simulink model "NPNV_CSAD_model"  (R2017a)
settings: Solver=ode4  StartTime=0.0  StopTime=t_sim  FixedStep=0.01  RelTol=1e-3
values from neighbouring files (symbols this model uses):
  eta_initial = [5; -1; 0]    [Run4corner.m]    (also in Simulation_plot.m = [-4; -2; 0.6*pi])
  gamma = 1.5    [Run4corner.m]
  nu_initial = [0; 0; 0]    [Run4corner.m]    (also in Simulation_plot.m)
  sigma = 2    [Run4corner.m]
undefined symbols (not defined in the file or in its folder): fdesignblkfcn, gcbh
libraries: simulink x4, dsparch4 x1
settings Model: Creator=torees  LastModifiedBy=torees

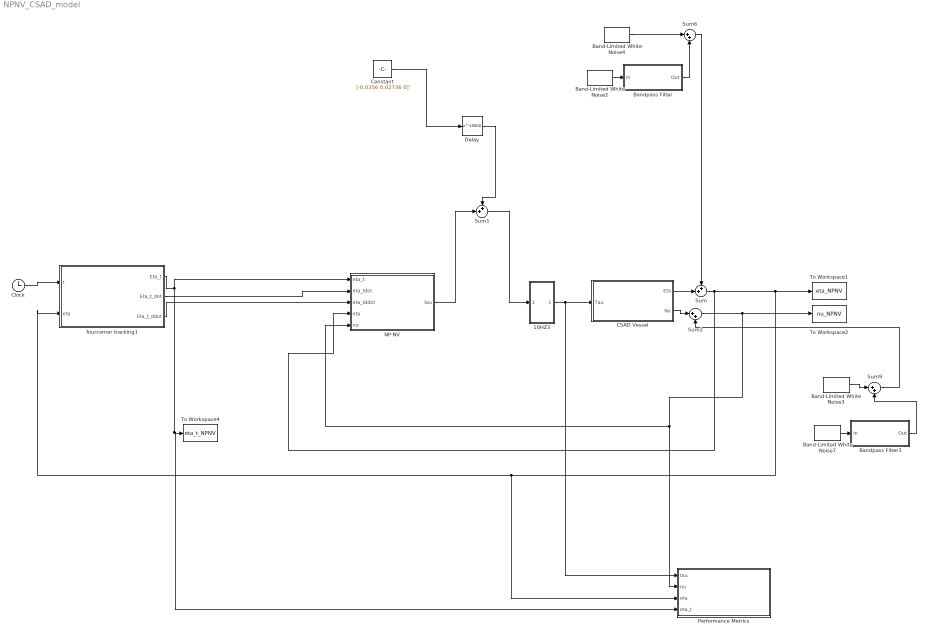
== system NPNV_CSAD_model ==
  10HZ3 : Subsystem
  Band-Limited White Noise2 : simulink/Sources/Band-Limited White Noise  Cov=posnoise  Ts=0.01  seed=[233451]
  Band-Limited White Noise3 : simulink/Sources/Band-Limited White Noise  Cov=velnoise2  Ts=0.01  seed=[233451]
  Band-Limited White Noise4 : simulink/Sources/Band-Limited White Noise  Cov=posnoise2  Ts=0.01  seed=[233451]
  Band-Limited White Noise7 : simulink/Sources/Band-Limited White Noise  Cov=velnoise  Ts=0.01  seed=[23345]
  Bandpass Filter : Subsystem  DialogController=fdesignblkfcn  InitFcn=fdesignblkfcn(gcbh, {'InitFcn'});  mask(Bandpass Filter){}
      mask help: Design a bandpass filter
      settings: CopyFcn=fdesignblkfcn(gcbh, {'CopyFcn'});
      mask Help: helpview(mapfilelocation('dsp'), 'dspbandpassfilter');
      mask Display: disp('Bandpass');
  Bandpass Filter3 : Subsystem  DialogController=fdesignblkfcn  InitFcn=fdesignblkfcn(gcbh, {'InitFcn'});  mask(Bandpass Filter){}
      mask help: Design a bandpass filter
      settings: CopyFcn=fdesignblkfcn(gcbh, {'CopyFcn'});
      mask Help: helpview(mapfilelocation('dsp'), 'dspbandpassfilter');
      mask Display: disp('Bandpass');
  CSAD Vessel : Subsystem
  Clock : Clock
  Constant : Constant  Value=[-0.0356 0.02736 0]'
  Delay : Delay  DelayLength=15000  InitialCondition=0
  NP-NV : Subsystem
  "Performance Metrics " : Subsystem
  Sum : Sum  Inputs=++|
  Sum1 : Sum  Inputs=++|
  Sum2 : Sum  Inputs=|++
  Sum6 : Sum  Inputs=|++
  Sum9 : Sum  Inputs=|++
  To Workspace1 : ToWorkspace  VariableName=eta_NPNV  SampleTime=-1
  To Workspace2 : ToWorkspace  VariableName=nu_NPNV  SampleTime=-1
  To Workspace4 : ToWorkspace  VariableName=eta_t_NPNV  SampleTime=-1
  fourcorner tracking1 : MATLAB Function  TreatAsAtomicUnit=on
  wires:
  Clock/1 -> fourcorner tracking1/1(t)
  Sum1/1 -> 10HZ3/1(In1)
  10HZ3/1(Out1) -> "Performance Metrics "/1(tau), CSAD Vessel/1(Tau)
  fourcorner tracking1/1(Eta_t) -> "Performance Metrics "/4(eta_t), To Workspace4/1, NP-NV/1(eta_t)
  fourcorner tracking1/2(Eta_t_dot) -> NP-NV/2(eta_tdot)
  fourcorner tracking1/3(Eta_t_ddot) -> NP-NV/3(eta_tddot)
  Sum6/1 -> Sum/1
  CSAD Vessel/1(Eta) -> Sum/2
  Sum/1 -> "Performance Metrics "/3(eta), fourcorner tracking1/2(eta), To Workspace1/1, NP-NV/4(eta)
  Delay/1 -> Sum1/1
  NP-NV/1(tau) -> Sum1/2
  CSAD Vessel/2(Nu) -> Sum2/1
  Sum9/1 -> Sum2/2
  Sum2/1 -> NP-NV/5(nu), "Performance Metrics "/2(nu), To Workspace2/1
  Constant/1 -> Delay/1
  Band-Limited White Noise2/1 -> Bandpass Filter/1(In)
  Band-Limited White Noise4/1 -> Sum6/1
  Bandpass Filter/1(Out) -> Sum6/2
  Bandpass Filter3/1(Out) -> Sum9/2
  Band-Limited White Noise3/1 -> Sum9/1
  Band-Limited White Noise7/1 -> Bandpass Filter3/1(In)

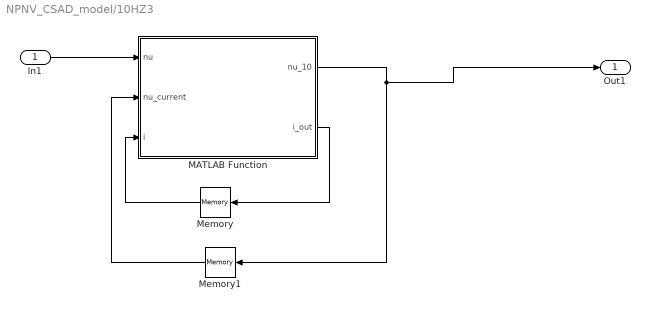
== system NPNV_CSAD_model/10HZ3 ==
  In1 : Inport
  MATLAB Function : MATLAB Function  TreatAsAtomicUnit=on
  Memory : Memory
  Memory1 : Memory
  Out1 : Outport
  wires:
  In1/1 -> MATLAB Function/1(nu)
  MATLAB Function/1(nu_10) -> Memory1/1, Out1/1
  Memory1/1 -> MATLAB Function/2(nu_current)
  MATLAB Function/2(i_out) -> Memory/1
  Memory/1 -> MATLAB Function/3(i)

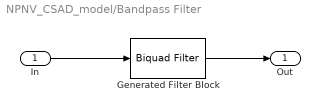
== system NPNV_CSAD_model/Bandpass Filter ==
  In : Inport
  Generated Filter Block : dsparch4/Biquad Filter  Tag=BlockMethodSubSystem  IIRFiltStruct=Direct form II  CoeffSource=Specify via dialog  BiQuadCoeffs=[0.28932621448050977 -0.19800857833013893 0.28932621448050977 1 -0.62679229449728924 0.99326477861490148;2 -1.1003519967587603 2 1 -0.60508947521969358 0.99323977127646146]  a0Flag=Warning  IC=0  ICnum=0  ICden=0  denAccumFracLength=30  denProdOutputFracLength=30  secondMemoryFracLength=15  roundingMode=Floor  overflowMode=off  ScaleValues=[0.0063942944592789474;1;8.4992509081585865]  optimizeScaleValues=off  ScaleValueMode=Specify via input port (g)  scaleValueFracLength=14  FilterSource=Specify via dialog  FilterObject=BQF
      settings: SourceProductName=DSP System Toolbox
  Out : Outport
  wires:
  In/1 -> Generated Filter Block/1
  Generated Filter Block/1 -> Out/1

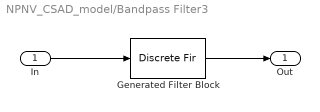
== system NPNV_CSAD_model/Bandpass Filter3 ==
  In : Inport
  Generated Filter Block : DiscreteFir  Tag=BlockMethodSubSystem  Coefficients=[-0.00079916321459414256 0.00032403449583075965 0.0011103641181887203 0.00036251169928540301 -0.0010006208701309827 -0.0010529558624241767 0.00042247970506665205 0.0014337707539335287 0.00046392998912194242 -0.0012699771729577363 -0.0013261148515873755 0.00052825480198556642 0.0017806682220775237 0.00057253310721010274 -0.0015579403216620623 -0.0016176685166059228 0.00064097161479369062 0.0021497454476688454 0.00068789900070729702 -0.0018633612906794794 -0.001926423966618558 0.00076015783376762245 0.0025394203872170606 0.00080952232829501457 -0.0021848742766087973 -0.0022509729150716933 0.00088525944440233741 0.0029478485691564844 0.00093681730481494862 -0.0025209046819104023 -0.0025897001978467645 0.0010156441843386106 0.0033729349354923851 0.0010691215618221929 -0.0028696797458744754 -0.0029407949247964556 0.0011506060003265994 0.003812348898990897 0.0012057009948789105 -0.0032292417393970374 -0.0033022641741789404 0.0012893704679716328 0.0042635424867300802 0.0013457555550174948 -0.0035974636052109902 -0.0036719491047843252 0.0014311011238421125 0.0047237713985051914 0.0014884259288208323 -0.0039720668915110471 -0.0040475433271385287 0.0015749066468750648 0.0051901187680907018 0.0016328010391898516 -0.0043506417948832978 -0.0044266133435287595 0.0017198488140888818 0.0056595213772874303 0.0017779262872743499 -0.0047306690985537492 -0.0048066208371846924 0.0018649511445690331 0.0061287980375845435 0.0019228124454002008 -0.0051095437646606241 -0.0051849465642018798 0.0020092081356957846 0.006594679822660582 0.0020664451012924151 -0.0054845999149232246 -0.0055589155781061344 0.0021515949867898466 0.0070538418073091422 0.00220779454561572 -0.0058531369131032737 -0.0059258234966891535 0.0022910776978809157 0.007502935945119746 0.0023458259879516803 -0.0062124462453399905 -0.0062829635042002249 0.0024266234252861554 0.0079386246987328078 0.0024795099809151538 -0.0065598388810737601 -0.0066276537694263263 0.0025572109712026269 0.0083576150230118152 0.0026078329282708682 -0.0068926727880481882 -0.0069572649518199582 0.002681841281647562 0.0087566922932573402 0.0027298075507009036 -0.007208380269975662 -0.0072692474638047866 0.0027995478258770264 0.0091327537677777949 0.0028444831823420526 -0.0075044947949431794 -0.0075611581577669394 0.0029094067308983286 0.0094828411767955405 0.0029509557723789931 -0.0077786769865693843 -0.0078306861110607664 0.0030105465468665557 0.0098041720378108516 0.0030483774688243128 -0.0080287394582629224 -0.0080756771915687642 0.0031021575230111413 0.010094169311068033 0.0031359656661302583 -0.0082526701835870051 -0.0082941570998561007 0.0031835002792112198 0.010350489027525429 0.0032130114043830301 -0.0084486541125467305 -0.0084843526015811205 0.0032539137653757461 0.010571045545472292 0.0032788870154664479 -0.0086150927643738641 -0.0086447106853366346 0.0033128224092882838 0.010754034120360252 0.0033330529206425396 -0.0087506215518108801 -0.0087739154062236469 0.0033597423634324232 0.010897950505146132 0.0033750634943581687 -0.0088541246196704986 -0.0088709022038571377 0.003394286772396473 0.011001607335037392 0.003404571920619809 -0.0089247470111965682 -0.008934869514801146 0.0034161699946112351 0.011064147090502434 0.0034213339808147739 -0.0089619040090547896 -0.0089652875331887021 0.003425210725237336 0.011085051475196808 0.003425210725237336 -0.0089652875331887021 -0.0089619040090547896 0.0034213339808147739 0.011064147090502434 0.0034161699946112351 -0.008934869514801146 -0.0089247470111965682 0.003404571920619809 0.011001607335037392 0.003394286772396473 -0.0088709022038571377 -0.0088541246196704986 0.0033750634943581687 0.010897950505146132 0.0033597423634324232 -0.0087739154062236469 -0.0087506215518108801 0.0033330529206425396 0.010754034120360252 0.0033128224092882838 -0.0086447106853366346 -0.0086150927643738641 0.0032788870154664479 0.010571045545472292 0.0032539137653757461 -0.0084843526015811205 -0.0084486541125467305 0.0032130114043830301 0.010350489027525429 0.0031835002792112198 ...(+2603 chars)]  InputProcessing=Columns as channels (frame based)
  Out : Outport
  wires:
  In/1 -> Generated Filter Block/1
  Generated Filter Block/1 -> Out/1

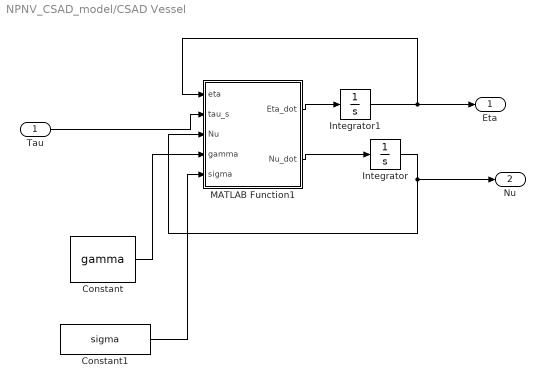
== system NPNV_CSAD_model/CSAD Vessel ==
  Tau : Inport
  Constant : Constant  Value=gamma
  Constant1 : Constant  Value=sigma
  Integrator : Integrator  InitialCondition=nu_initial
  Integrator1 : Integrator  InitialCondition=eta_initial
  MATLAB Function1 : MATLAB Function  TreatAsAtomicUnit=on
  Eta : Outport
  Nu : Outport  Port=2
  wires:
  Integrator/1 -> Nu/1, MATLAB Function1/3(Nu)
  MATLAB Function1/1(Eta_dot) -> Integrator1/1
  Integrator1/1 -> Eta/1, MATLAB Function1/1(eta)
  MATLAB Function1/2(Nu_dot) -> Integrator/1
  Tau/1 -> MATLAB Function1/2(tau_s)
  Constant1/1 -> MATLAB Function1/5(sigma)
  Constant/1 -> MATLAB Function1/4(gamma)

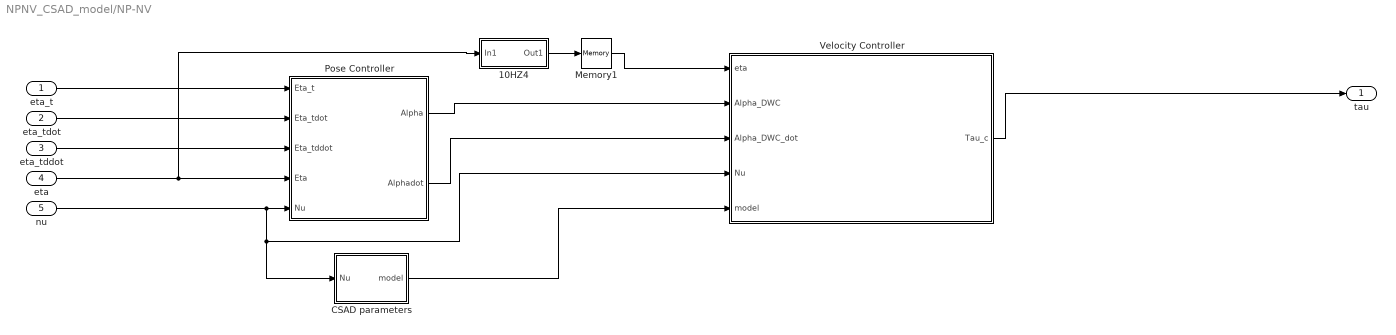
== system NPNV_CSAD_model/NP-NV ==
  eta_t : Inport
  eta_tdot : Inport  Port=2
  eta_tddot : Inport  Port=3
  eta : Inport  Port=4
  nu : Inport  Port=5
  " Pose Controller" : MATLAB Function  TreatAsAtomicUnit=on
  10HZ4 : Subsystem
  CSAD parameters : MATLAB Function  TreatAsAtomicUnit=on
  Memory1 : Memory  X0=[ 0 0 0]'
  Velocity Controller : MATLAB Function  TreatAsAtomicUnit=on
  tau : Outport
  wires:
  eta_t/1 -> " Pose Controller"/1(Eta_t)
  eta_tdot/1 -> " Pose Controller"/2(Eta_tdot)
  eta_tddot/1 -> " Pose Controller"/3(Eta_tddot)
  eta/1 -> 10HZ4/1(In1), " Pose Controller"/4(Eta)
  nu/1 -> Velocity Controller/4(Nu), CSAD parameters/1(Nu), " Pose Controller"/5(Nu)
  CSAD parameters/1(model) -> Velocity Controller/5(model)
  " Pose Controller"/2(Alphadot) -> Velocity Controller/3(Alpha_DWC_dot)
  " Pose Controller"/1(Alpha) -> Velocity Controller/2(Alpha_DWC)
  Velocity Controller/1(Tau_c) -> tau/1
  10HZ4/1(Out1) -> Memory1/1
  Memory1/1 -> Velocity Controller/1(eta)

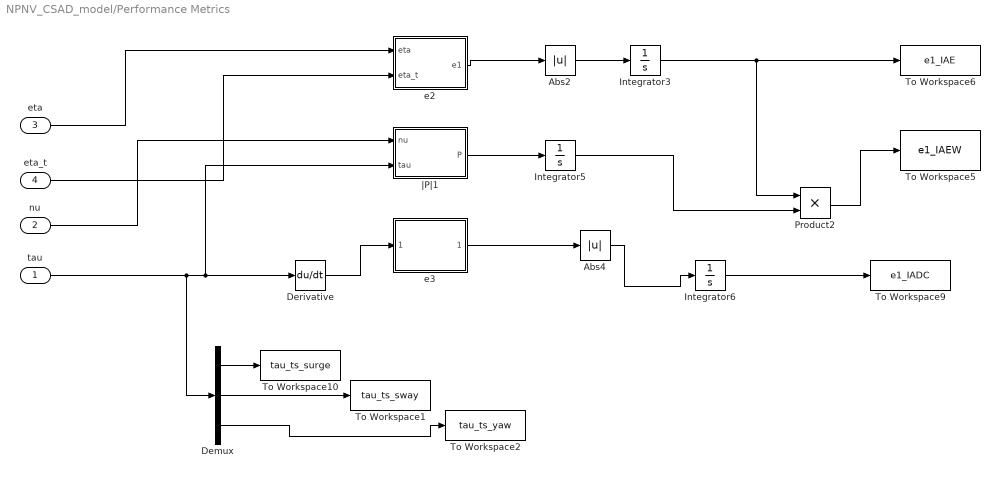
== system NPNV_CSAD_model/Performance Metrics  ==
  tau : Inport
  nu : Inport  Port=2
  eta : Inport  Port=3
  eta_t : Inport  Port=4
  Abs2 : Abs
  Abs4 : Abs
  Demux : Demux  Outputs=3
  Derivative : Derivative
  Integrator3 : Integrator
  Integrator5 : Integrator
  Integrator6 : Integrator
  Product2 : Product
  To Workspace1 : ToWorkspace  VariableName=tau_ts_sway  SaveFormat=Timeseries  SampleTime=-1
  To Workspace10 : ToWorkspace  VariableName=tau_ts_surge  SaveFormat=Timeseries  SampleTime=-1
  To Workspace2 : ToWorkspace  VariableName=tau_ts_yaw  SaveFormat=Timeseries  SampleTime=-1
  To Workspace5 : ToWorkspace  VariableName=e1_IAEW  SaveFormat=Timeseries  SampleTime=-1
  To Workspace6 : ToWorkspace  VariableName=e1_IAE  SaveFormat=Timeseries  SampleTime=-1
  To Workspace9 : ToWorkspace  VariableName=e1_IADC  SaveFormat=Timeseries  SampleTime=-1
  e2 : MATLAB Function  TreatAsAtomicUnit=on
  e3 : MATLAB Function  TreatAsAtomicUnit=on
  |P|1 : MATLAB Function  TreatAsAtomicUnit=on
  wires:
  eta_t/1 -> e2/2(eta_t)
  eta/1 -> e2/1(eta)
  nu/1 -> |P|1/1(nu)
  tau/1 -> Demux/1, |P|1/2(tau), Derivative/1
  Integrator3/1 -> Product2/1, To Workspace6/1
  |P|1/1(P) -> Integrator5/1
  e2/1(e1) -> Abs2/1
  e3/1(tau_dot) -> Abs4/1
  Abs2/1 -> Integrator3/1
  Derivative/1 -> e3/1(tau_dot_in)
  Integrator6/1 -> To Workspace9/1
  Integrator5/1 -> Product2/2
  Product2/1 -> To Workspace5/1
  Abs4/1 -> Integrator6/1
  Demux/1 -> To Workspace10/1
  Demux/2 -> To Workspace1/1
  Demux/3 -> To Workspace2/1

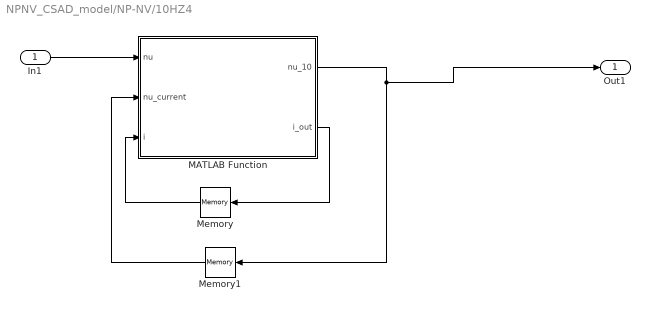
== system NPNV_CSAD_model/NP-NV/10HZ4 ==
  In1 : Inport
  MATLAB Function : MATLAB Function  TreatAsAtomicUnit=on
  Memory : Memory
  Memory1 : Memory
  Out1 : Outport
  wires:
  In1/1 -> MATLAB Function/1(nu)
  MATLAB Function/1(nu_10) -> Memory1/1, Out1/1
  Memory1/1 -> MATLAB Function/2(nu_current)
  MATLAB Function/2(i_out) -> Memory/1
  Memory/1 -> MATLAB Function/3(i)

== matlab function NPNV_CSAD_model/NP-NV/CSAD parameters ==
  data: model output; Nu input
function model = fcn(Nu)

X_u		= -5.35;		
X_uu 	=  0;		
X_uuu	= -19.6312;

Y_v		= -10.16;   
Y_vv	= -0.8647;
Y_vvv	= -681.1745;	

Y_r		= -7.25;
Y_rr	= -3.45;
Y_rrr   = 0;

N_v		= 0;		
N_vv	= -0.2088;
N_vvv = 0;

N_r		= -14.55;
N_rr	= -9.9597;
N_rrr	= -0.3101;

N_rv	= 0.08;	
N_vr	= 0.08;
Y_rv	= -0.805;			
Y_vr	= -0.845;

X_ud =     -10;
Y_vd =     -105;
Y_rd =     -0.525;
N_vd =     -0.157;	
N_rd =     -3.4950;

Nur  = -Y_rd;
Nuv  = -(Y_vd-X_ud);
Yur  = -X_ud;

x_g     = 0.0375;
m       = 127.92;
I_z     = 61.967;

u   = Nu(1);
v   = Nu(2);
r   = Nu(3);

d_11 = - X_u - X_uu*abs(u) - X_uuu*u^2;
d_22 = - Y_v - Y_vv*abs(v) - Y_rv*abs(r) - Y_vvv*v^2;
d_23 = - Y_r - Y_rr*abs(r) - Y_vr*abs(v) - Y_rrr*r^2 - Yur*u;
d_32 = - N_v - N_vv*abs(v) - N_rv*abs(r) - N_vvv*v^2 - Nuv*u;
d_33 = - N_r - N_rr*abs(r) - N_vr*abs(v) - N_rrr*r^2 - Nur*u;

D    = [d_11  0     0
        0     d_22  d_23
        0     d_32  d_33];

CA=[0                            0          Y_vd*v+Y_rd*r;
    0                            0                -X_ud*u;
    -Y_rd*r-Y_vd*v               X_ud*u                0];

CRB=[0             0     -m*(x_g*r+v);
     0             0      m*u;
     m*(x_g*r+v) -m*u     0]; 

C=CRB+CA;

M_RB_c=[m     0      0;
        0     m      m*x_g;
        0     m*x_g  I_z];

M_A_c=[-X_ud    0      0;
         0    -Y_vd  -Y_rd;
         0    -N_vd  -N_rd];     
    
M = M_RB_c + M_A_c;

model=[M C D];

== matlab function NPNV_CSAD_model/fourcorner tracking1 ==
  data: t input; Eta_t output; Eta_t_dot output; Eta_t_ddot output; eta input
function [ Eta_t, Eta_t_dot, Eta_t_ddot]   =  fourcorner_tracking(t,eta)

v_t = 0.15;

etaP = [5 7 7 7 5 5;
       -1 -1 1 1 1 -1;
        0 0 0 pi/4 pi/4 0];
Eta_t_dot = [0;0;0];
Eta_t_ddot = [0;0;0];

Eta_t = [5;-1;0];
persistent point ;
if(isempty(point))
    point = 1;
    
end


switch point
    case 1
        Eta_t = etaP(:,2);
         if ((abs((Eta_t(1)- eta(1))) <0.01 ) ==1  ) && ((abs(Eta_t(2)-eta(2))<0.01) ==1) && (abs(Eta_t(3)-rad2deg(eta(3)))<3 == 1)
            point = 2;
            return;
         end
        
        
    case 2
        Eta_t = etaP(:,3);
        if((abs((Eta_t(1)- eta(1))) <0.01 ) ==1  ) && ((abs(Eta_t(2)-eta(2))<0.01) ==1) && (abs(Eta_t(3)-rad2deg(eta(3)))<3 == 1) 
            point = 3;
            return;
         end
    case 3
        Eta_t = etaP(:,4);
        if((abs((Eta_t(1)- eta(1))) <0.01 ) ==1  ) && ((abs(Eta_t(2)-eta(2))<0.01) ==1) && (rad2deg(abs(Eta_t(3)-eta(3)))<3 == 1)  
            point = 4;
            return;
            
         end
    case 4
        Eta_t = etaP(:,5);
        if((abs((Eta_t(1)- eta(1))) <0.01 ) ==1  ) && ((abs(Eta_t(2)-eta(2))<0.01) ==1) && (rad2deg(abs(Eta_t(3)-eta(3)))<3 == 1) 
            point = 5; 
            return;
         end
    case 5
        Eta_t = etaP(:,6);
        if((abs((Eta_t(1)- eta(1))) <0.01 ) ==1  ) && ((abs(Eta_t(2)-eta(2))<0.01) ==1) && (abs(Eta_t(3)-rad2deg(eta(3)))<3 == 1) 
            point = 6;          
            return;
         end

    otherwise
        

end
end
%(abs(Eta_t(2)-eta(2))<0.01) &&

== matlab function NPNV_CSAD_model/NP-NV/Velocity Controller ==
  data: eta input; Alpha_DWC input; Alpha_DWC_dot input; Tau_c output; Nu input; model input
function Tau_c = VelocityControl(eta,Alpha_DWC, Alpha_DWC_dot,Nu,model)

M = model(1:3,1:3);
C = model(1:3,4:6);
D = model(1:3,7:9);

z2 = Nu - Alpha_DWC;
psi=eta(3);
Gamma2 = diag([0.2,0.2 , 0.1745])*M;
delta_v = 0.7;
delta_r = 1;

z2_v = [z2(1), z2(2)]';
z2_r = z2(3);

first = 1/(sqrt(z2_v'*z2_v + delta_v^2));
second = 1/(sqrt(z2_r^2 + delta_r^2));

K2 = Gamma2*[first*eye(2,2) zeros(2,1); zeros(1,2) second];

z2 = Nu - Alpha_DWC;


R_T = [cos(psi) -sin(psi) 0;
       sin(psi) cos(psi) 0;
       0 0 1]';







%linear model
Tau_c = M * Alpha_DWC_dot + C*Alpha_DWC+ D * Alpha_DWC - K2 * z2 ;


end

== matlab function NPNV_CSAD_model/NP-NV/ Pose Controller ==
  data: Eta_t input; Eta_tdot input; Eta_tddot input; Eta input; Nu input; Alpha output; Alphadot output
function [ Alpha ,Alphadot]  = PoseControl(Eta_t, Eta_tdot,Eta_tddot, Eta, Nu)
Gamma1 =  diag([0.08, 0.08, 0.0697]);
delta_psi = 0.5;
delta_p = 0.5;

psi = Eta(3);
r = Nu(3);

S = [0 -r  0; r  0  0; 0  0  0];
S_T = S';
R = [cos(psi) -sin(psi) 0; sin(psi) cos(psi) 0; 0 0 1];
R_T = R';

z1 = R_T * (Eta - Eta_t);

z1_p = [z1(1), z1(2)]';
z1_psi = z1(3);

first = 1/(sqrt(z1_p'*z1_p + delta_p^2));
second = 1/(sqrt(z1_psi^2 + delta_psi^2));

K1 = Gamma1*[first*eye(2,2) zeros(2,1); zeros(1,2) second];

Nu_d = R_T * Eta_tdot - K1 * z1;
Alpha = Nu_d;
z2 = Nu - Alpha;

z1dot = S_T * z1 - K1 * z1 + z2;

z1_p = [z1(1), z1(2)]';
z1_psi = z1(3);
z1_pdot = [z1dot(1), z1dot(2)]';
z1_psidot = z1dot(3);

first2 = (z1_p'*z1_pdot)/((z1_p'*z1_p + delta_p^2)^(3/2));

second2 = (z1_psi*z1_psidot)/((z1_psi^2 + delta_psi^2)^(3/2));

K1dot = - Gamma1*[first2*eye(2,2) zeros(2,1); zeros(1,2) second2];

Alphadot = R_T * Eta_tddot + S_T * R_T * Eta_tdot - K1dot * z1 - K1*z1dot;

end

== matlab function NPNV_CSAD_model/Performance Metrics /e2 ==
  data: e1 output; eta input; eta_t input
function e1 = fcn(eta,eta_t)

x = eta(1);
y = eta(2);
psi = eta(3);

x_t = eta_t(1);
y_t = eta_t(2);
psi_t = eta_t(3);

x_tilde = x-x_t;
y_tilde = y-y_t;
psi_tilde = psi-psi_t;

e1 = sqrt((x_tilde^2)/4 + (y_tilde^2)/4 + (psi_tilde^2)/(pi/2));

== matlab function NPNV_CSAD_model/NP-NV/10HZ4/MATLAB Function ==
  data: nu input; nu_10 output; nu_current input; i input; i_out output
function [nu_10,i_out] = hz(nu,nu_current,i)

if i==0
    nu_10=nu;
    i_out=1;
elseif i==10
    nu_10=nu;
    i_out=1;
else
    nu_10=nu_current;
    i_out=i+1;
end

== matlab function NPNV_CSAD_model/Performance Metrics /e3 ==
  data: tau_dot output; tau_dot_in input
function tau_dot = fcn(tau_dot_in)

tau1 = tau_dot_in(1);
tau2 = tau_dot_in(2);
tau3 = tau_dot_in(3);



tau_dot = sqrt((tau1^2) + (tau2^2) + (tau3^2));

== matlab function NPNV_CSAD_model/Performance Metrics /|P|1 ==
  data: nu input; P output; tau input
function P  = fcn(nu, tau)
P = abs(nu'*tau);

== matlab function NPNV_CSAD_model/10HZ3/MATLAB Function ==
  data: nu input; nu_10 output; nu_current input; i input; i_out output
function [nu_10,i_out] = hz(nu,nu_current,i)

if i==0
    nu_10=nu;
    i_out=1;
elseif i==10
    nu_10=nu;
    i_out=1;
else
    nu_10=nu_current;
    i_out=i+1;
end

== matlab function NPNV_CSAD_model/CSAD Vessel/MATLAB Function1 ==
  data: eta input; tau_s input; Eta_dot output; Nu input; Nu_dot output; gamma input; sigma input
function [Eta_dot,Nu_dot] = Vessel(eta,tau_s,Nu,gamma,sigma)

Nu_dot = CSAD_full(Nu,tau_s,gamma,sigma);

yaw = eta(3);

R =[cos(yaw) -sin(yaw) 0;
            sin(yaw)  cos(yaw) 0;
            0         0        1]; 
Eta_dot = R*Nu;
end
